simulink model "Controller_Step_11"  (Simulink 7.9)
settings: Solver=FixedStepDiscrete  StartTime=0.0  StopTime=100  FixedStep=0.5  MaxStep=1  RelTol=1e-3
PostLoadFcn:
  | m = 150;
  | load mybus
libraries: simulink x1
settings Model: Creator=wcampbel  LastModifiedBy=wcampbel
settings DataIOCC: SaveOutput=off  SaveTime=off
settings OptimizationCC: BlockReduction=off  ConditionallyExecuteInputs=off  InlineParams=on  OptimizeModelRefInitCode=on
settings DebuggingCC: FcnCallInpInsideContextMsg=Use local settings  StrictBusMsg=Warning
settings SFSimCC: SimParseCustomCode=off
settings RTWCC: SystemTargetFile=ert.tlc  GenCodeOnly=on  GenerateMakefile=off  TemplateMakefile=ert_default_tmf  Description=Real-Time Workshop Embedded Coder  GenerateReport=on  RTWVerbose=off  ProcessScript=ert_make_rtw_hook  IncludeHyperlinkInReport=on  LaunchReport=on  GenerateTraceInfo=on  GenerateTraceReport=on  GenerateTraceReportSl=on  GenerateTraceReportSf=on  GenerateTraceReportEml=on
settings CodeAppCC: IgnoreCustomStorageClasses=off  SimulinkDataObjDesc=on  SFDataObjDesc=on  CustomSymbolStrGlobalVar=$N$M  CustomSymbolStrBlkIO=$N$M  InsertBlockDesc=on  ReqsInCode=on
settings ERTTargetCC: CodeReplacementLibrary=ANSI_C  MultiwordLength=2048  IncludeMdlTerminateFcn=off  SupportAbsoluteTime=off  SupportNonFinite=off  SupportComplex=off  InlinedParameterPlacement=NonHierarchical  ERTCustomFileTemplate=example_file_process.tlc  ConvertIfToSwitch=off  SuppressUnreachableDefaultCases=off

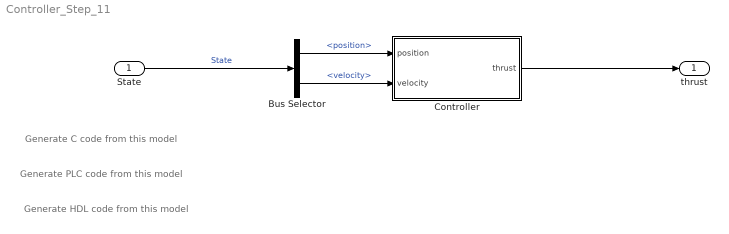
== system Controller_Step_11 ==
  note: Generate PLC code from this model
  note: Generate HDL code from this model
  note: Generate C code from this model
  State : Inport  Description=This variable defines the state of a vehicle under controlled descent. The first element is position in meters. The second is velocity in meters per second.  OutDataTypeStr=Bus: stateBus
  Bus Selector : BusSelector  OutputSignals=position,velocity
  Controller : Subsystem  TreatAsAtomicUnit=on
  thrust : Outport  OutDataTypeStr=double  PortDimensions=3
  wires:
  Controller/1(thrust) -> thrust/1
  State/1 -> Bus Selector/1  "State"
  Bus Selector/1 -> Controller/1(position)  "<position>"
  Bus Selector/2 -> Controller/2(velocity)  "<velocity>"

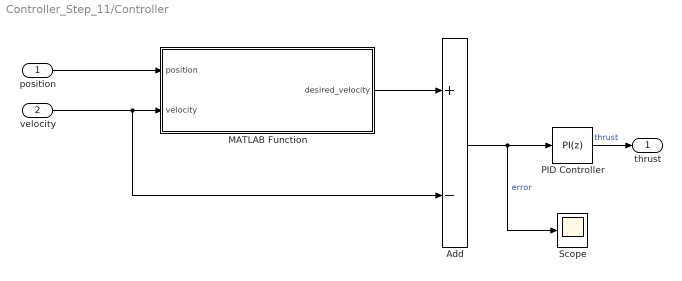
== system Controller_Step_11/Controller ==
  position : Inport
  velocity : Inport  Port=2
  Add : Sum  Inputs=+-
  MATLAB Function : MATLAB Function  TreatAsAtomicUnit=on
  PID Controller : simulink/Continuous/PID Controller  Controller=PI  TimeDomain=Discrete-time  SampleTime=0.5  IntegratorMethod=Forward Euler  FilterMethod=Forward Euler  Form=Parallel  P=50  I=5  D=0  N=100  InitialConditionSource=internal  InitialConditionForIntegrator=0  InitialConditionForFilter=0  ExternalReset=none  LimitOutput=on  UpperSaturationLimit=2000  LowerSaturationLimit=0  LinearizeAsGain=off  AntiWindupMode=none  Kb=1  TrackingMode=off  Kt=1  PParamMin=[]  PParamMax=[]  IParamMin=[]  IParamMax=[]  DParamMin=[]  DParamMax=[]  NParamMin=[]  NParamMax=[]  KbParamMin=[]  KbParamMax=[]  KtParamMin=[]  KtParamMax=[]  POutMin=[]  POutMax=[]  IOutMin=[]  IOutMax=[]  DOutMin=[]  DOutMax=[]  NOutMin=[]  NOutMax=[]  KbOutMin=[]  KbOutMax=[]  KtOutMin=[]  KtOutMax=[]  IntegratorOutMin=[]  IntegratorOutMax=[]  FilterOutMin=[]  FilterOutMax=[]  SumOutMin=[]  SumOutMax=[]  SumI1OutMin=[]  SumI1OutMax=[]  SumI2OutMin=[]  SumI2OutMax=[]  SumI3OutMin=[]  SumI3OutMax=[]  SumDOutMin=[]  SumDOutMax=[]  SaturationOutMin=[]  SaturationOutMax=[]  IntegratorContinuousStateAttributes=''  IntegratorStateMustResolveToSignalObject=off  IntegratorRTWStateStorageClass=Auto  FilterContinuousStateAttributes=''  FilterStateMustResolveToSignalObject=off  FilterRTWStateStorageClass=Auto
  Scope : Scope
      settings: ShowLegends=on  TimeRange=27.56653992395438  YMin=-10  YMax=19.90625
  thrust : Outport
  wires:
  MATLAB Function/1(desired_velocity) -> Add/1
  Add/1 -> PID Controller/1, Scope/1  "error"
  position/1 -> MATLAB Function/1(position)
  velocity/1 -> MATLAB Function/2(velocity), Add/2
  PID Controller/1 -> thrust/1  "thrust"

== matlab function Controller/MATLAB Function ==
  data: position input double; desired_velocity output double; velocity input double
function desired_velocity = variable_v(position,velocity)

height = position(3);

if height > 500
   desired_descent_rate = velocity(3);
elseif height > 200
   desired_descent_rate = -10;
elseif height > 100
   desired_descent_rate = -2;
elseif height > 10
   desired_descent_rate = -1;
else
   desired_descent_rate = -0.5;
end

desired_velocity = [0; 0; desired_descent_rate];
